simulink model "LQR_ship"  (R2023b)
settings: Solver=VariableStepAuto  StartTime=0.0  StopTime=tf  RelTol=1e-6
values from neighbouring files (symbols this model uses):
  A = Ixx-Kpdot    (= 4100300)    [ShipFinStabilizers.m]
  A_lin = [0, 1; (D+E)/A, B/A]    [ShipFinStabilizers.m]    (also in plotRoutine.m = [0, 1; d+e, b])
  B = Kp + Kup - 2*Kalpha*rf/U    (= -505089.3115)    [ShipFinStabilizers.m]
  B_lin = [0; F/A]    [ShipFinStabilizers.m]    (also in plotRoutine.m = [0; f])
  C = Knl    (= -416000)    [ShipFinStabilizers.m]
  C_lin = [180/pi,0]    [ShipFinStabilizers.m]    (also in plotRoutine.m = [180/pi, 0])
  controller_on = 0    [off.m]    (also in on.m = 1; plotRoutine.m)
  D = KphiUU*U^2    (= -265500)    [ShipFinStabilizers.m]
  F = -2*Kalpha    (= -18034.875)    [ShipFinStabilizers.m]
  Fw = 0    [ShipFinStabilizers.m]    (also in plotRoutine.m = 0.1)
  lin_sim = 0    [ShipFinStabilizers.m]    (also in plotRoutine.m)
  omega_w = 0.3    [ShipFinStabilizers.m]    (also in plotRoutine.m = 1.3)
  sat = 45    [ShipFinStabilizers.m]
  x0 = [deg2rad(10);0]    [ShipFinStabilizers.m]    (also in plotRoutine.m)
settings Model: Creator=valen  LastModifiedBy=valen

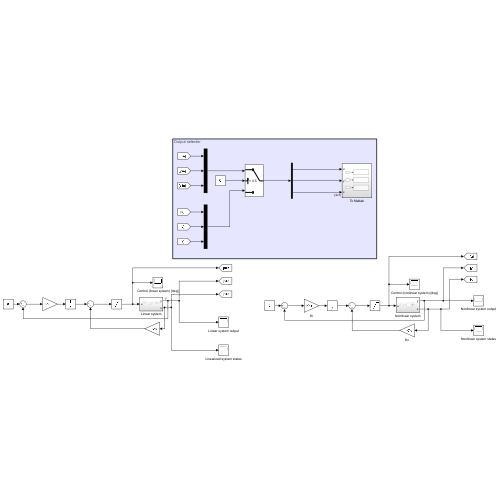
[thumbnail: Simulink's stored preview of the top-level diagram]
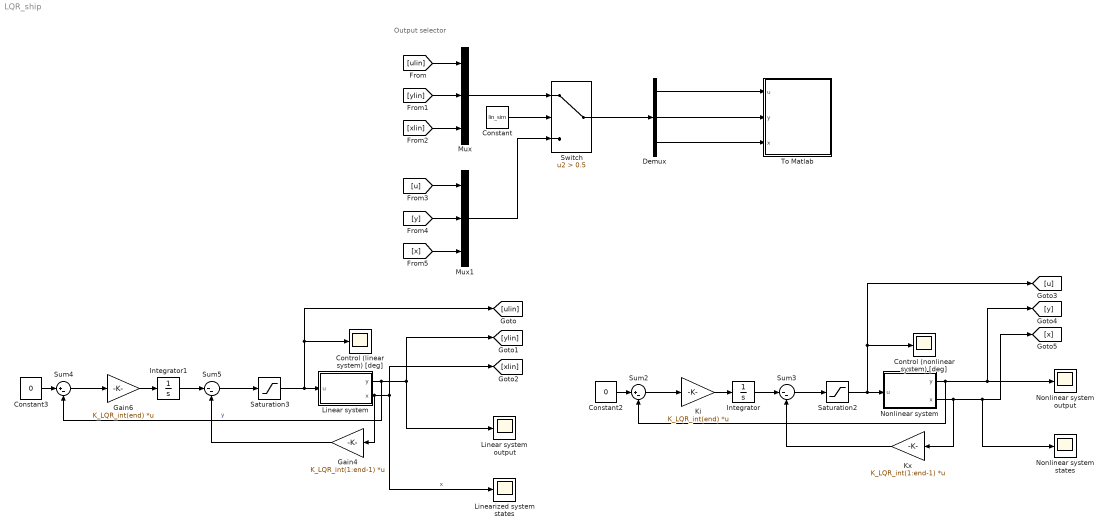
== system LQR_ship ==
  note: Output selector
  Constant : Constant  Value=lin_sim
  Constant2 : Constant  Value=0
  Constant3 : Constant  Value=0
  Control (linear system) [deg] : Scope
  Control (nonlinear system) [deg] : Scope
  Demux : Demux  Outputs=3
  Gain4 : Gain  Gain=K_LQR_int(1:end-1)  Multiplication=Matrix(K*u)
  Gain6 : Gain  Gain=K_LQR_int(end)  Multiplication=Matrix(K*u)
  Integrator : Integrator
  Integrator1 : Integrator
  Ki : Gain  Gain=K_LQR_int(end)  Multiplication=Matrix(K*u)
  Kx : Gain  Gain=K_LQR_int(1:end-1)  Multiplication=Matrix(K*u)
  Linear system : Subsystem
  Linear system output : Scope
  Linearized system states : Scope
  Mux : Mux  Inputs=3
  Mux1 : Mux  Inputs=3
  Nonlinear system : Subsystem
  Nonlinear system output : Scope
  Nonlinear system states : Scope
  Saturation2 : Saturate  UpperLimit=sat  LowerLimit=-sat
  Saturation3 : Saturate  UpperLimit=sat  LowerLimit=-sat
  Sum2 : Sum  Inputs=|+-
  Sum3 : Sum  Inputs=|--
  Sum4 : Sum  Inputs=|+-
  Sum5 : Sum  Inputs=|--
  Switch : Switch  Criteria=u2 > Threshold  Threshold=0.5  SaturateOnIntegerOverflow=off  InputSameDT=off
  To Matlab : Subsystem
  wires:
  Constant2/1 -> Sum2/1
  Nonlinear system/1(y) -> [y], Nonlinear system output/1, Sum2/2
  Integrator/1 -> Sum3/1
  Sum3/1 -> Saturation2/1
  Nonlinear system/2(x) -> [x], Nonlinear system states/1, Kx/1
  Kx/1 -> Sum3/2
  Gain4/1 -> Sum5/2
  Integrator1/1 -> Sum5/1
  Sum4/1 -> Gain6/1
  Constant3/1 -> Sum4/1
  Linear system/2(x) -> [xlin], Linearized system states/1, Gain4/1  "x"
  Linear system/1(y) -> [ylin], Linear system output/1, Sum4/2  "y"
  Sum5/1 -> Saturation3/1
  Gain6/1 -> Integrator1/1
  Ki/1 -> Integrator/1
  Sum2/1 -> Ki/1
  Demux/1 -> To Matlab/1(u)
  Demux/2 -> To Matlab/2(y)
  Demux/3 -> To Matlab/3(x)
  Switch/1 -> Demux/1
  Mux/1 -> Switch/1
  Constant/1 -> Switch/2
  [x] -> Mux1/3
  Mux1/1 -> Switch/3
  [u] -> Mux1/1
  [xlin] -> Mux/3
  [y] -> Mux1/2
  [ulin] -> Mux/1
  [ylin] -> Mux/2
  Saturation3/1 -> [ulin], Control (linear system) [deg]/1, Linear system/1(u)
  Saturation2/1 -> Nonlinear system/1(u), [u], Control (nonlinear system) [deg]/1

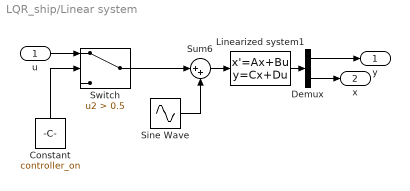
== system LQR_ship/Linear system ==
  u : Inport
  Constant : Constant  Value=controller_on
  Demux : Demux  Outputs=[1,2]
  Linearized system1 : StateSpace  A=A_lin  B=B_lin  C=[C_lin;eye(2)]  D=[0;0;0]  InitialCondition=x0
  Sine Wave : Sin  Amplitude=Fw/F*A  Frequency=omega_w  SampleTime=0
  Sum6 : Sum  Inputs=|++
  Switch : Switch  Criteria=u2 > Threshold  Threshold=0.5  SaturateOnIntegerOverflow=off  InputSameDT=off
  y : Outport
  x : Outport  Port=2
  wires:
  Sum6/1 -> Linearized system1/1
  Linearized system1/1 -> Demux/1
  Demux/1 -> y/1
  Demux/2 -> x/1
  Sine Wave/1 -> Sum6/2
  u/1 -> Switch/1
  Constant/1 -> Switch/2
  Switch/1 -> Sum6/1

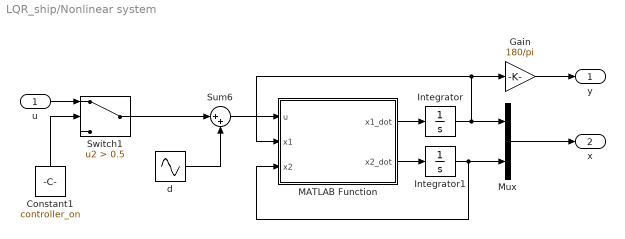
== system LQR_ship/Nonlinear system ==
  u : Inport
  Constant1 : Constant  Value=controller_on
  Gain : Gain  Gain=180/pi
  Integrator : Integrator  InitialCondition=x0(1)
  Integrator1 : Integrator  InitialCondition=x0(2)
  MATLAB Function : MATLAB Function  TreatAsAtomicUnit=on
  Mux : Mux  Inputs=2
  Sum6 : Sum  Inputs=|++
  Switch1 : Switch  Criteria=u2 > Threshold  Threshold=0.5  SaturateOnIntegerOverflow=off  InputSameDT=off
  d : Sin  Amplitude=Fw/F*A  Frequency=omega_w  SampleTime=0
  y : Outport
  x : Outport  Port=2
  wires:
  Integrator1/1 -> Mux/2, MATLAB Function/3(x2)
  Integrator/1 -> Mux/1, Gain/1, MATLAB Function/2(x1)
  MATLAB Function/2(x2_dot) -> Integrator1/1
  MATLAB Function/1(x1_dot) -> Integrator/1
  Mux/1 -> x/1
  Sum6/1 -> MATLAB Function/1(u)
  Gain/1 -> y/1
  Constant1/1 -> Switch1/2
  u/1 -> Switch1/1
  d/1 -> Sum6/2
  Switch1/1 -> Sum6/1

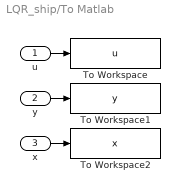
== system LQR_ship/To Matlab ==
  u : Inport  PortDimensions=1
  y : Inport  Port=2  PortDimensions=1
  x : Inport  Port=3  PortDimensions=[2,1]
  To Workspace : ToWorkspace  VariableName=u  SaveFormat=Structure With Time  SampleTime=-1
  To Workspace1 : ToWorkspace  VariableName=y  SaveFormat=Structure With Time  SampleTime=-1
  To Workspace2 : ToWorkspace  VariableName=x  SaveFormat=Structure With Time  SampleTime=-1
  wires:
  u/1 -> To Workspace/1
  x/1 -> To Workspace2/1
  y/1 -> To Workspace1/1

== matlab function LQR_ship/Nonlinear system/MATLAB Function ==
  data: u input; x1_dot output; x1 input; x2 input; x2_dot output; A parameter; B parameter; C parameter; D parameter; E parameter; F parameter
function [x1_dot,x2_dot] = ship(u,x1,x2, A, B, C, D, E, F)

    x1_dot = x2;
    x2_dot = 1/A*( B*x2 + C*x2*abs(x2) + D*x1 + E*sin(x1) + F*u);
